simulink model "Exercise_charging_stateflow"  (R2024b)
settings: Solver=ode3  StartTime=0.0  StopTime=30.0  FixedStep=1  RelTol=1e-3
libraries: simulink x2
settings Model: Creator=balaj  LastModifiedBy=balaj

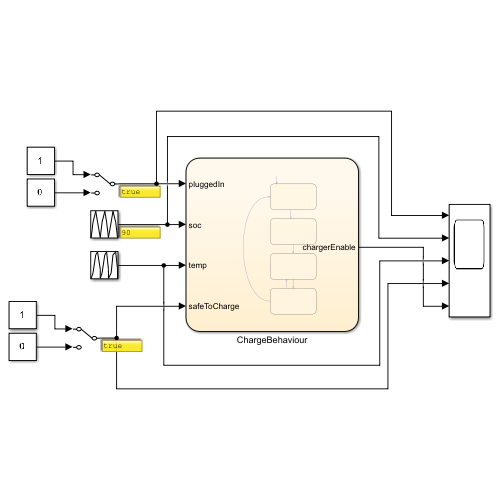
[thumbnail: Simulink's stored preview of the top-level diagram]
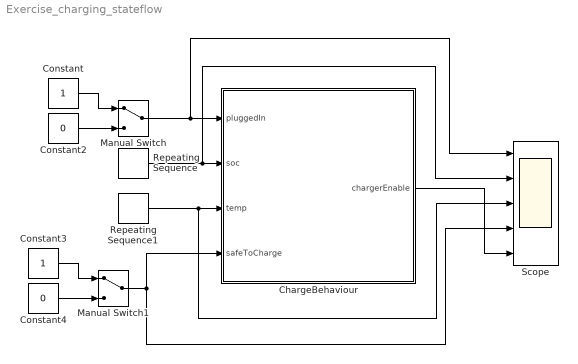
== system Exercise_charging_stateflow ==
  ChargeBehaviour : Stateflow chart  TreatAsAtomicUnit=on
  Constant : Constant  OutDataTypeStr=boolean
  Constant2 : Constant  Value=0  OutDataTypeStr=boolean
  Constant3 : Constant  OutDataTypeStr=boolean
  Constant4 : Constant  Value=0  OutDataTypeStr=boolean
  Manual Switch : ManualSwitch
  Manual Switch1 : ManualSwitch
  Repeating Sequence : simulink/Sources/Repeating Sequence  rep_seq_t=[0 5 10 15 20]  rep_seq_y=[20 60 90 60 20]
  Repeating Sequence1 : simulink/Sources/Repeating Sequence  rep_seq_t=[0 5 10 15 20]  rep_seq_y=[5 15 45 50 20]
  Scope : Scope  NumInputPorts=5
  wires:
  Manual Switch/1 -> Scope/1, ChargeBehaviour/1(pluggedIn)
  Repeating Sequence/1 -> Scope/2, ChargeBehaviour/2(soc)
  Repeating Sequence1/1 -> Scope/3, ChargeBehaviour/3(temp)
  Manual Switch1/1 -> Scope/4, ChargeBehaviour/4(safeToCharge)
  ChargeBehaviour/1(chargerEnable) -> Scope/5
  Constant/1 -> Manual Switch/1
  Constant2/1 -> Manual Switch/2
  Constant3/1 -> Manual Switch1/1
  Constant4/1 -> Manual Switch1/2

== stateflow chart Exercise_charging_stateflow/ChargeBehaviour ==
  state Idle
    entry:
    chargerEnable=0;
  state PreCharge
    entry:
    chargerEnable=0;
  state Charging
    entry:
    chargerEnable=1;
  state Cutoff
    entry:
    chargerEnable=0;
  (default) -> Idle
  Cutoff -> Idle [order 1] : [pluggedIn==0]
  Idle -> PreCharge : [pluggedIn==1]
  PreCharge -> Charging : [safeToCharge==1]
  Cutoff -> Charging [order 2] : [soc<25 && pluggedIn==1 && safeToCharge==1]
  Charging -> Cutoff : [soc>=80 || temp>=45]
  data: pluggedIn input boolean; soc input double; temp input double; safeToCharge input boolean; chargerEnable output
